simulink model "Task1_version5"  (R2021a)
settings: Solver=FixedStepAuto  StartTime=0.0  StopTime=0.05  FixedStep=1e-7  MaxStep=1e-7  RelTol=1e-3
values from neighbouring files (symbols this model uses):
  f0 = str2double(inputStr)    [PWM.m]
  fs = Switching_frequency(j)    [PWM.m]
  M = 1    [PWM.m]
  Mode = 1    [PWM.m]
libraries: simulink x4, spspowerguiLib x1
settings Model: OrderedModelArguments=off  Creator=es-mostafamoh111  LastModifiedBy=es-mostafamoh111
settings DataIOCC: ReturnWorkspaceOutputs=off

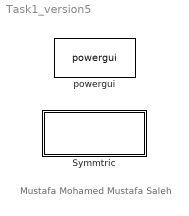
== system Task1_version5 ==
  note: Mustafa Mohamed Mustafa Saleh
  Symmtric : Subsystem
  powergui : spspowerguiLib/powergui  Priority=1  SimulationMode=Discrete  SampleTime=1e-7  frequency=60  Iterations=50  frequencyindice=0  Pbase=100e6  ErrMax=1e-4  UnitsV=kV  UnitsW=MW  buscounter=0  FunctionMessages=off  echomessages=off  EnableUseOfTLC=off  CurrentSourceSwitches=off  DisableSnubberDevices=off  DisableRonSwitches=off  DisableVfSwitches=off  DisplayEquations=off  AutomaticDiscreteSolvers=off  SolverType=Tustin/Backward Euler (TBE)  Interpol=off  ExternalGateDelay=off  methode=off  Ts=100  x0status=blocks  SPID=on  SwTol=0  HookPort=off  NonlinearTolerance=1e-4  nMaxIteration=100  ContinueOnMaxIteration=off  RestoreLinks=warning  ResistiveCurrentMeasurement=off  Frange=[0:2:500]  Ylog=off  Xlog=on  ShowGrid=off  save=off  variable=ZData  structure=0  ZoomFFT=off  StartTime=0.0  cycles=1  DisplayStyle=1  fundamental=60  FreqAxis=off  MaxFrequency=1000  frequencyindicesteady=1  RmsSteady=1  display=off

== system Task1_version5/Symmtric ==
  Symmetric DPWM1 : Subsystem
  Symmetric SPWM : Subsystem
  Symmetric SVM : Subsystem

== system Task1_version5/Symmtric/Symmetric DPWM1 ==
  DPWM max : Subsystem  Commented=on  TreatAsAtomicUnit=on
  DPWM min : Subsystem  Commented=on  TreatAsAtomicUnit=on
  DPWM1 : Subsystem
  Nature sine DPWM : Subsystem  Commented=on

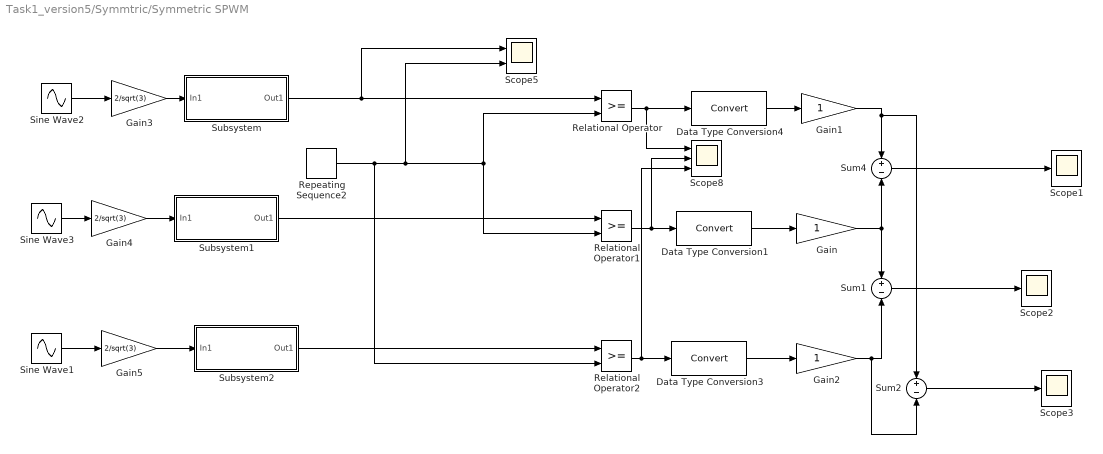
== system Task1_version5/Symmtric/Symmetric SPWM ==
  Data Type Conversion1 : DataTypeConversion
  Data Type Conversion3 : DataTypeConversion
  Data Type Conversion4 : DataTypeConversion
  Gain : Gain
  Gain1 : Gain  OutDataTypeStr=Inherit: Inherit via back propagation
  Gain2 : Gain
  Gain3 : Gain  Gain=2/sqrt(3)
  Gain4 : Gain  Gain=2/sqrt(3)
  Gain5 : Gain  Gain=2/sqrt(3)
  Relational Operator : RelationalOperator  OutDataTypeStr=boolean  RndMeth=Simplest
  Relational Operator1 : RelationalOperator  OutDataTypeStr=boolean  RndMeth=Simplest
  Relational Operator2 : RelationalOperator  OutDataTypeStr=boolean  RndMeth=Simplest
  Repeating Sequence2 : simulink/Sources/Repeating Sequence  rep_seq_t=[0 1/(4*fs) 2/(4*fs) 3/(4*fs) 1/fs ]  rep_seq_y=[1 0 -1 0 1]
  Scope1 : Scope
  Scope2 : Scope
  Scope3 : Scope
  Scope5 : Scope  NumInputPorts=2
  Scope8 : Scope  NumInputPorts=3
  Sine Wave1 : Sin  Amplitude=M  Frequency=f0*2*pi  Phase=2*pi/3  SampleTime=0
  Sine Wave2 : Sin  Amplitude=M  Frequency=f0*2*pi  SampleTime=0
  Sine Wave3 : Sin  Amplitude=M  Frequency=f0*2*pi  Phase=-2*pi/3  SampleTime=0
  Subsystem : Subsystem
  Subsystem1 : Subsystem
  Subsystem2 : Subsystem
  Sum1 : Sum  Inputs=+-
  Sum2 : Sum  Inputs=+-
  Sum4 : Sum  Inputs=+-
  wires:
  Gain/1 -> Sum4/2, Sum1/1
  Gain1/1 -> Sum2/1, Sum4/1
  Repeating Sequence2/1 -> Relational Operator2/2, Scope5/2, Relational Operator/2, Relational Operator1/2
  Subsystem/1(Out1) -> Scope5/1, Relational Operator/1
  Sine Wave2/1 -> Gain3/1
  Relational Operator1/1 -> Scope8/2, Data Type Conversion1/1
  Relational Operator/1 -> Scope8/1, Data Type Conversion4/1
  Sine Wave1/1 -> Gain5/1
  Data Type Conversion3/1 -> Gain2/1
  Relational Operator2/1 -> Scope8/3, Data Type Conversion3/1
  Data Type Conversion4/1 -> Gain1/1
  Data Type Conversion1/1 -> Gain/1
  Gain2/1 -> Sum2/2, Sum1/2
  Sine Wave3/1 -> Gain4/1
  Subsystem1/1(Out1) -> Relational Operator1/1
  Subsystem2/1(Out1) -> Relational Operator2/1
  Sum4/1 -> Scope1/1
  Sum1/1 -> Scope2/1
  Sum2/1 -> Scope3/1
  Gain3/1 -> Subsystem/1(In1)
  Gain4/1 -> Subsystem1/1(In1)
  Gain5/1 -> Subsystem2/1(In1)

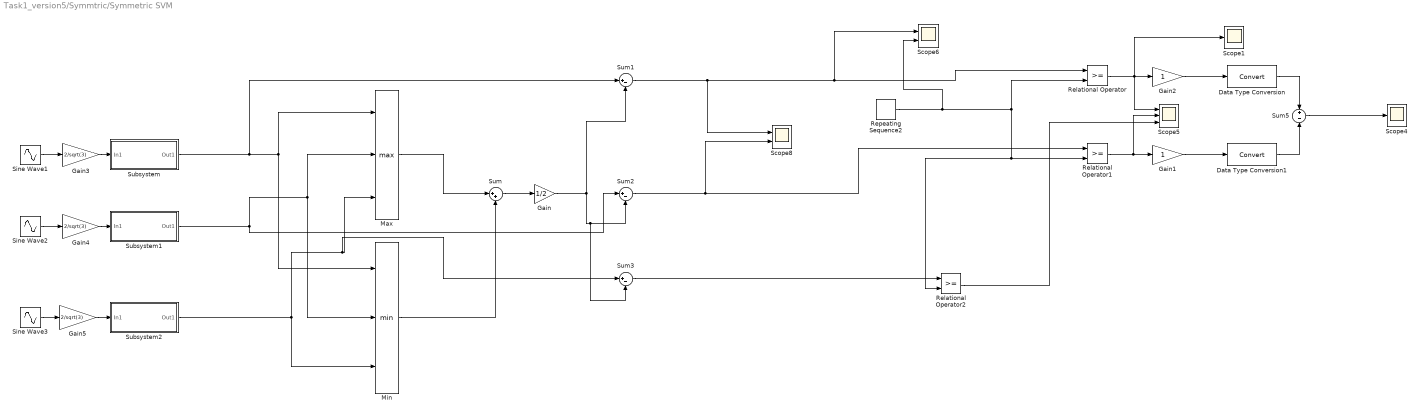
== system Task1_version5/Symmtric/Symmetric SVM ==
  Data Type Conversion : DataTypeConversion
  Data Type Conversion1 : DataTypeConversion
  Gain : Gain  Gain=1/2
  Gain1 : Gain
  Gain2 : Gain
  Gain3 : Gain  Gain=2/sqrt(3)
  Gain4 : Gain  Gain=2/sqrt(3)
  Gain5 : Gain  Gain=2/sqrt(3)
  Max : MinMax  Function=max  Inputs=3
  Min : MinMax  Inputs=3
  Relational Operator : RelationalOperator  OutDataTypeStr=boolean  RndMeth=Simplest
  Relational Operator1 : RelationalOperator  OutDataTypeStr=boolean  RndMeth=Simplest
  Relational Operator2 : RelationalOperator  OutDataTypeStr=boolean  RndMeth=Simplest
  Repeating Sequence2 : simulink/Sources/Repeating Sequence  rep_seq_t=[0 1/(4*fs) 2/(4*fs) 3/(4*fs) 1/fs ]  rep_seq_y=[1 0 -1 0 1]
  Scope1 : Scope
  Scope4 : Scope
  Scope5 : Scope  NumInputPorts=3
  Scope6 : Scope  NumInputPorts=2
  Scope8 : Scope  NumInputPorts=2
  Sine Wave1 : Sin  Amplitude=M  Frequency=f0*2*pi  SampleTime=0
  Sine Wave2 : Sin  Amplitude=M  Frequency=f0*2*pi  Phase=-2*pi/3  SampleTime=0
  Sine Wave3 : Sin  Amplitude=M  Frequency=f0*2*pi  Phase=2*pi/3  SampleTime=0
  Subsystem : Subsystem
  Subsystem1 : Subsystem
  Subsystem2 : Subsystem
  Sum : Sum  Inputs=|++
  Sum1 : Sum  Inputs=|+-
  Sum2 : Sum  Inputs=|+-
  Sum3 : Sum  Inputs=|+-
  Sum5 : Sum  Inputs=+-
  wires:
  Subsystem/1(Out1) -> Sum1/1, Min/1, Max/1
  Relational Operator/1 -> Scope1/1, Gain2/1, Scope5/1
  Repeating Sequence2/1 -> Scope6/2, Relational Operator/2, Relational Operator1/2, Relational Operator2/2
  Sum/1 -> Gain/1
  Subsystem1/1(Out1) -> Min/2, Max/2, Sum2/1
  Relational Operator1/1 -> Scope5/2, Gain1/1
  Gain/1 -> Sum2/2, Sum3/2, Sum1/2
  Max/1 -> Sum/1
  Gain1/1 -> Data Type Conversion1/1
  Min/1 -> Sum/2
  Data Type Conversion1/1 -> Sum5/2
  Data Type Conversion/1 -> Sum5/1
  Gain2/1 -> Data Type Conversion/1
  Subsystem2/1(Out1) -> Sum3/1, Max/3, Min/3
  Relational Operator2/1 -> Scope5/3
  Sum3/1 -> Relational Operator2/1
  Sum2/1 -> Relational Operator1/1, Scope8/2
  Sum1/1 -> Scope6/1, Relational Operator/1, Scope8/1
  Sine Wave1/1 -> Gain3/1
  Sine Wave2/1 -> Gain4/1
  Sine Wave3/1 -> Gain5/1
  Sum5/1 -> Scope4/1
  Gain3/1 -> Subsystem/1(In1)
  Gain4/1 -> Subsystem1/1(In1)
  Gain5/1 -> Subsystem2/1(In1)

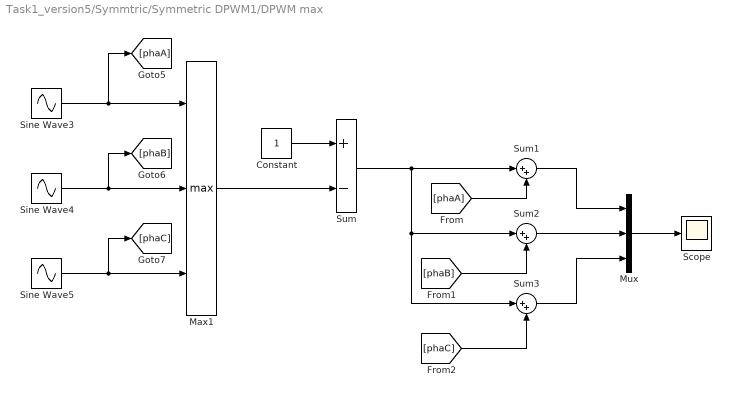
== system Task1_version5/Symmtric/Symmetric DPWM1/DPWM max ==
  Constant : Constant
  Max1 : MinMax  Function=max  Inputs=3
  Mux : Mux  Inputs=3
  Scope : Scope
  Sine Wave3 : Sin  Frequency=2*pi*f0  SampleTime=0
  Sine Wave4 : Sin  Frequency=2*pi*f0  Phase=-2*pi/3  SampleTime=0
  Sine Wave5 : Sin  Frequency=2*pi*f0  Phase=2*pi/3  SampleTime=0
  Sum : Sum  Inputs=+-
  Sum1 : Sum  Inputs=|++
  Sum2 : Sum  Inputs=|++
  Sum3 : Sum  Inputs=|++
  wires:
  Sine Wave4/1 -> [phaB], Max1/2
  Sine Wave3/1 -> [phaA], Max1/1
  Sine Wave5/1 -> [phaC], Max1/3
  [phaB] -> Sum2/2
  Sum/1 -> Sum2/1, Sum3/1, Sum1/1
  Sum3/1 -> Mux/3
  Sum1/1 -> Mux/1
  Sum2/1 -> Mux/2
  Mux/1 -> Scope/1
  [phaA] -> Sum1/2
  [phaC] -> Sum3/2
  Constant/1 -> Sum/1
  Max1/1 -> Sum/2

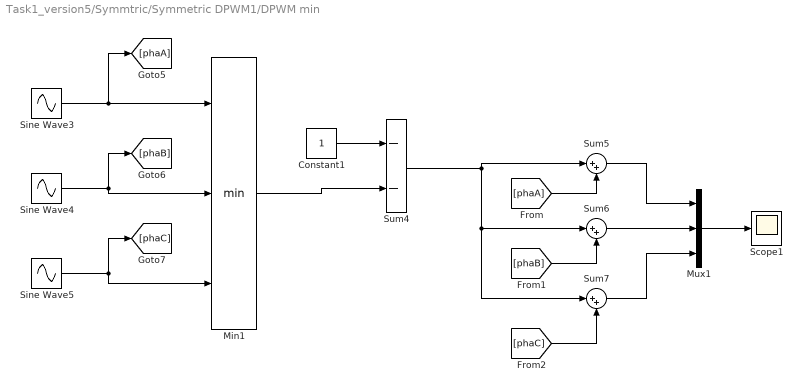
== system Task1_version5/Symmtric/Symmetric DPWM1/DPWM min ==
  Constant1 : Constant
  Min1 : MinMax  Inputs=3
  Mux1 : Mux  Inputs=3
  Scope1 : Scope
  Sine Wave3 : Sin  Frequency=2*pi*f0  SampleTime=0
  Sine Wave4 : Sin  Frequency=2*pi*f0  Phase=-2*pi/3  SampleTime=0
  Sine Wave5 : Sin  Frequency=2*pi*f0  Phase=2*pi/3  SampleTime=0
  Sum4 : Sum  Inputs=--
  Sum5 : Sum  Inputs=|++
  Sum6 : Sum  Inputs=|++
  Sum7 : Sum  Inputs=|++
  wires:
  Min1/1 -> Sum4/2
  Sine Wave4/1 -> [phaB], Min1/2
  Sine Wave3/1 -> [phaA], Min1/1
  Sine Wave5/1 -> [phaC], Min1/3
  [phaA] -> Sum5/2
  [phaB] -> Sum6/2
  Mux1/1 -> Scope1/1
  Sum7/1 -> Mux1/3
  [phaC] -> Sum7/2
  Sum5/1 -> Mux1/1
  Sum6/1 -> Mux1/2
  Constant1/1 -> Sum4/1
  Sum4/1 -> Sum5/1, Sum6/1, Sum7/1

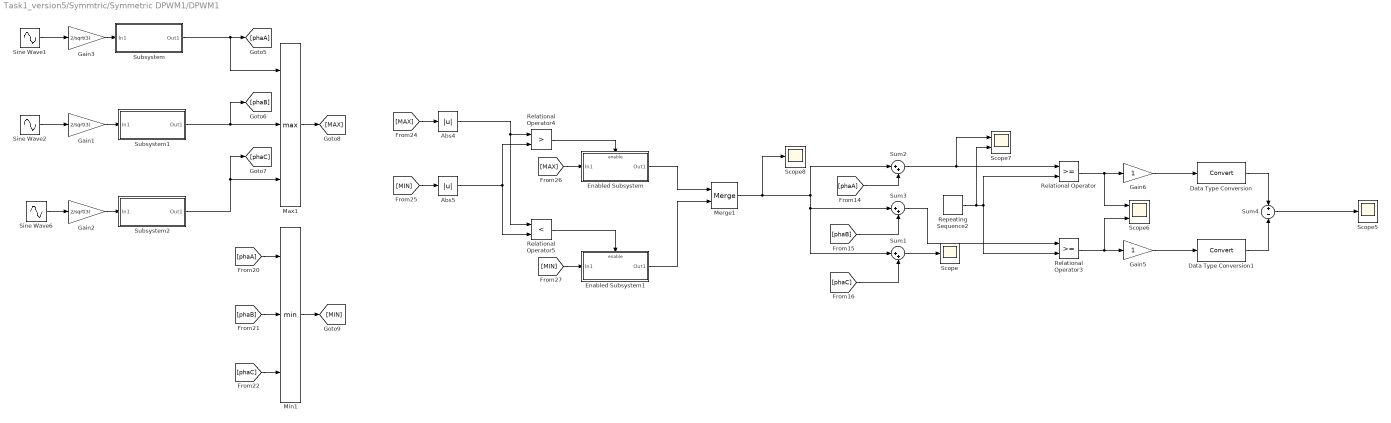
== system Task1_version5/Symmtric/Symmetric DPWM1/DPWM1 ==
  Abs4 : Abs
  Abs5 : Abs
  Data Type Conversion : DataTypeConversion
  Data Type Conversion1 : DataTypeConversion
  Enabled Subsystem : Subsystem  TreatAsAtomicUnit=on
  Enabled Subsystem1 : Subsystem  TreatAsAtomicUnit=on
  Gain1 : Gain  Gain=2/sqrt(3)
  Gain2 : Gain  Gain=2/sqrt(3)
  Gain3 : Gain  Gain=2/sqrt(3)
  Gain5 : Gain
  Gain6 : Gain
  Max1 : MinMax  Function=max  Inputs=3
  Merge1 : Merge
  Min1 : MinMax  Inputs=3
  Relational Operator : RelationalOperator  OutDataTypeStr=boolean  RndMeth=Simplest
  Relational Operator3 : RelationalOperator  OutDataTypeStr=boolean  RndMeth=Simplest
  Relational Operator4 : RelationalOperator  Operator=>  OutDataTypeStr=boolean  RndMeth=Simplest
  Relational Operator5 : RelationalOperator  Operator=<  OutDataTypeStr=boolean  RndMeth=Simplest
  Repeating Sequence2 : simulink/Sources/Repeating Sequence  rep_seq_t=[0 1/(4*fs) 2/(4*fs) 3/(4*fs) 1/fs ]  rep_seq_y=[1 0 -1 0 1]
  Scope : Scope
  Scope5 : Scope
  Scope6 : Scope  NumInputPorts=2
  Scope7 : Scope  NumInputPorts=2
  Scope8 : Scope
  Sine Wave1 : Sin  Amplitude=M  Frequency=f0*2*pi  SampleTime=0
  Sine Wave2 : Sin  Amplitude=M  Frequency=f0*2*pi  Phase=-2*pi/3  SampleTime=0
  Sine Wave6 : Sin  Amplitude=M  Frequency=f0*2*pi  Phase=2*pi/3  SampleTime=0
  Subsystem : Subsystem
  Subsystem1 : Subsystem
  Subsystem2 : Subsystem
  Sum1 : Sum  Inputs=|++
  Sum2 : Sum  Inputs=|++
  Sum3 : Sum  Inputs=|++
  Sum4 : Sum  Inputs=+-
  wires:
  Sine Wave1/1 -> Gain3/1
  Sine Wave6/1 -> Gain2/1
  Sine Wave2/1 -> Gain1/1
  Max1/1 -> [MAX]
  [MAX] -> Abs4/1
  [phaB] -> Min1/2
  Subsystem/1(Out1) -> Max1/1, [phaA]
  Min1/1 -> [MIN]
  [phaA] -> Min1/1
  [MIN] -> Enabled Subsystem1/1(In1)
  Abs5/1 -> Relational Operator5/2, Relational Operator4/2
  Subsystem2/1(Out1) -> [phaC], Max1/3
  [phaB] -> Sum3/2
  [phaC] -> Min1/3
  Subsystem1/1(Out1) -> [phaB], Max1/2
  Relational Operator4/1 -> Enabled Subsystem/Enable
  Enabled Subsystem1/1(Out1) -> Merge1/2
  Merge1/1 -> Sum2/1, Sum3/1, Sum1/1, Scope8/1
  Abs4/1 -> Relational Operator4/1, Relational Operator5/1
  [phaC] -> Sum1/2
  [MAX] -> Enabled Subsystem/1(In1)
  Enabled Subsystem/1(Out1) -> Merge1/1
  Relational Operator5/1 -> Enabled Subsystem1/Enable
  [MIN] -> Abs5/1
  [phaA] -> Sum2/2
  Repeating Sequence2/1 -> Scope7/2, Relational Operator/2, Relational Operator3/2
  Gain5/1 -> Data Type Conversion1/1
  Data Type Conversion1/1 -> Sum4/2
  Relational Operator3/1 -> Scope6/2, Gain5/1
  Gain6/1 -> Data Type Conversion/1
  Data Type Conversion/1 -> Sum4/1
  Relational Operator/1 -> Gain6/1, Scope6/1
  Sum2/1 -> Scope7/1, Relational Operator/1
  Sum3/1 -> Relational Operator3/1
  Sum1/1 -> Scope/1
  Sum4/1 -> Scope5/1
  Gain3/1 -> Subsystem/1(In1)
  Gain1/1 -> Subsystem1/1(In1)
  Gain2/1 -> Subsystem2/1(In1)

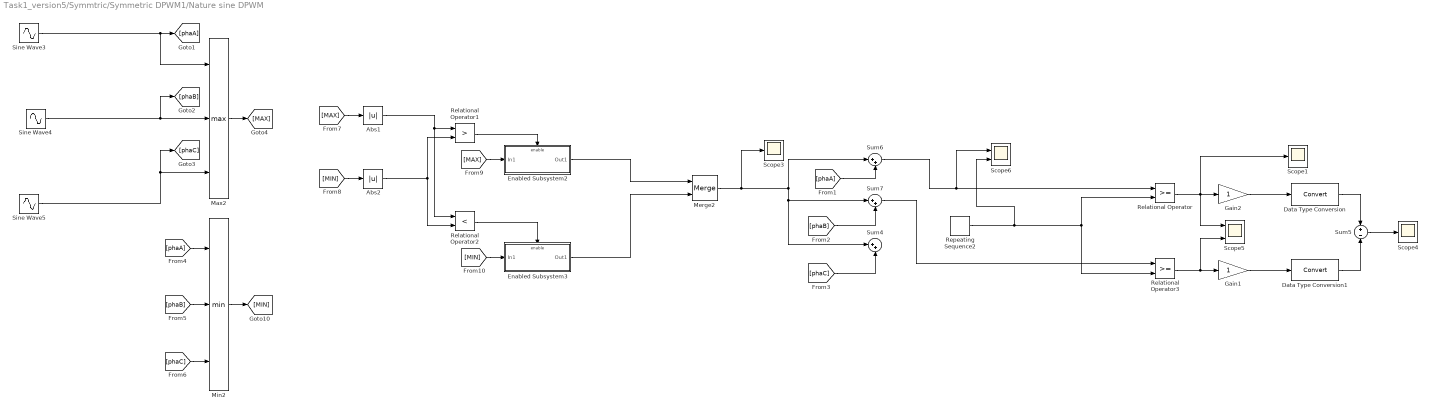
== system Task1_version5/Symmtric/Symmetric DPWM1/Nature sine DPWM ==
  Abs1 : Abs
  Abs2 : Abs
  Data Type Conversion : DataTypeConversion
  Data Type Conversion1 : DataTypeConversion
  Enabled Subsystem2 : Subsystem  TreatAsAtomicUnit=on
  Enabled Subsystem3 : Subsystem  TreatAsAtomicUnit=on
  Gain1 : Gain
  Gain2 : Gain
  Max2 : MinMax  Function=max  Inputs=3
  Merge2 : Merge
  Min2 : MinMax  Inputs=3
  Relational Operator : RelationalOperator  OutDataTypeStr=boolean  RndMeth=Simplest
  Relational Operator1 : RelationalOperator  Operator=>  OutDataTypeStr=boolean  RndMeth=Simplest
  Relational Operator2 : RelationalOperator  Operator=<  OutDataTypeStr=boolean  RndMeth=Simplest
  Relational Operator3 : RelationalOperator  OutDataTypeStr=boolean  RndMeth=Simplest
  Repeating Sequence2 : simulink/Sources/Repeating Sequence  rep_seq_t=[0 1/(4*fs) 2/(4*fs) 3/(4*fs) 1/fs ]  rep_seq_y=[1 0 -1 0 1]
  Scope1 : Scope
  Scope3 : Scope
  Scope4 : Scope
  Scope5 : Scope  NumInputPorts=2
  Scope6 : Scope  NumInputPorts=2
  Sine Wave3 : Sin  Amplitude=M  Frequency=f0*2*pi  SampleTime=0
  Sine Wave4 : Sin  Amplitude=M  Frequency=f0*2*pi  Phase=-2*pi/3  SampleTime=0
  Sine Wave5 : Sin  Amplitude=M  Frequency=f0*2*pi  Phase=2*pi/3  SampleTime=0
  Sum4 : Sum  Inputs=|++
  Sum5 : Sum  Inputs=+-
  Sum6 : Sum  Inputs=|++
  Sum7 : Sum  Inputs=|++
  wires:
  Abs2/1 -> Relational Operator2/2, Relational Operator1/2
  Min2/1 -> [MIN]
  Sine Wave5/1 -> [phaC], Max2/3
  [phaA] -> Min2/1
  Sine Wave4/1 -> [phaB], Max2/2
  [MIN] -> Enabled Subsystem3/1(In1)
  Sine Wave3/1 -> [phaA], Max2/1
  Merge2/1 -> Sum6/1, Sum7/1, Sum4/1, Scope3/1
  [phaC] -> Min2/3
  Enabled Subsystem3/1(Out1) -> Merge2/2
  Relational Operator2/1 -> Enabled Subsystem3/Enable
  Relational Operator1/1 -> Enabled Subsystem2/Enable
  Enabled Subsystem2/1(Out1) -> Merge2/1
  [phaB] -> Sum7/2
  [phaC] -> Sum4/2
  [MAX] -> Abs1/1
  [MAX] -> Enabled Subsystem2/1(In1)
  Abs1/1 -> Relational Operator1/1, Relational Operator2/1
  [phaA] -> Sum6/2
  [MIN] -> Abs2/1
  [phaB] -> Min2/2
  Max2/1 -> [MAX]
  Data Type Conversion/1 -> Sum5/1
  Gain2/1 -> Data Type Conversion/1
  Relational Operator3/1 -> Scope5/2, Gain1/1
  Sum5/1 -> Scope4/1
  Repeating Sequence2/1 -> Scope6/2, Relational Operator/2, Relational Operator3/2
  Relational Operator/1 -> Scope1/1, Gain2/1, Scope5/1
  Data Type Conversion1/1 -> Sum5/2
  Gain1/1 -> Data Type Conversion1/1
  Sum6/1 -> Scope6/1, Relational Operator/1
  Sum7/1 -> Relational Operator3/1

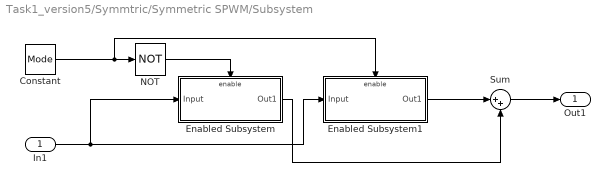
== system Task1_version5/Symmtric/Symmetric SPWM/Subsystem ==
  In1 : Inport
  Constant : Constant  Value=Mode
  Enabled Subsystem : Subsystem  TreatAsAtomicUnit=on
  Enabled Subsystem1 : Subsystem  TreatAsAtomicUnit=on
  NOT : Logic  Operator=NOT  IconShape=distinctive  AllPortsSameDT=off  OutDataTypeStr=boolean
  Sum : Sum  Inputs=|++
  Out1 : Outport
  wires:
  In1/1 -> Enabled Subsystem1/1(Input), Enabled Subsystem/1(Input)
  Constant/1 -> NOT/1, Enabled Subsystem1/Enable
  NOT/1 -> Enabled Subsystem/Enable
  Enabled Subsystem1/1(Out1) -> Sum/1
  Enabled Subsystem/1(Out1) -> Sum/2
  Sum/1 -> Out1/1

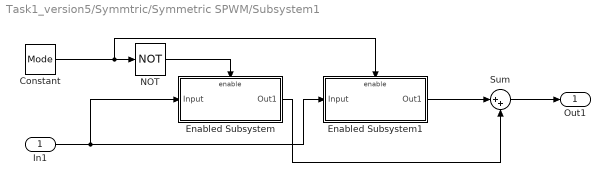
== system Task1_version5/Symmtric/Symmetric SPWM/Subsystem1 ==
  In1 : Inport
  Constant : Constant  Value=Mode
  Enabled Subsystem : Subsystem  TreatAsAtomicUnit=on
  Enabled Subsystem1 : Subsystem  TreatAsAtomicUnit=on
  NOT : Logic  Operator=NOT  IconShape=distinctive  AllPortsSameDT=off  OutDataTypeStr=boolean
  Sum : Sum  Inputs=|++
  Out1 : Outport
  wires:
  Sum/1 -> Out1/1
  Enabled Subsystem/1(Out1) -> Sum/2
  Enabled Subsystem1/1(Out1) -> Sum/1
  NOT/1 -> Enabled Subsystem/Enable
  Constant/1 -> Enabled Subsystem1/Enable, NOT/1
  In1/1 -> Enabled Subsystem/1(Input), Enabled Subsystem1/1(Input)

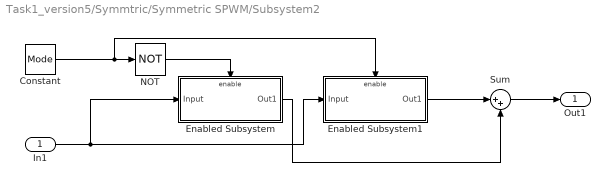
== system Task1_version5/Symmtric/Symmetric SPWM/Subsystem2 ==
  In1 : Inport
  Constant : Constant  Value=Mode
  Enabled Subsystem : Subsystem  TreatAsAtomicUnit=on
  Enabled Subsystem1 : Subsystem  TreatAsAtomicUnit=on
  NOT : Logic  Operator=NOT  IconShape=distinctive  AllPortsSameDT=off  OutDataTypeStr=boolean
  Sum : Sum  Inputs=|++
  Out1 : Outport
  wires:
  In1/1 -> Enabled Subsystem1/1(Input), Enabled Subsystem/1(Input)
  Constant/1 -> NOT/1, Enabled Subsystem1/Enable
  NOT/1 -> Enabled Subsystem/Enable
  Enabled Subsystem1/1(Out1) -> Sum/1
  Enabled Subsystem/1(Out1) -> Sum/2
  Sum/1 -> Out1/1

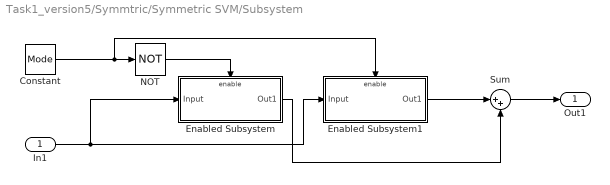
== system Task1_version5/Symmtric/Symmetric SVM/Subsystem ==
  In1 : Inport
  Constant : Constant  Value=Mode
  Enabled Subsystem : Subsystem  TreatAsAtomicUnit=on
  Enabled Subsystem1 : Subsystem  TreatAsAtomicUnit=on
  NOT : Logic  Operator=NOT  IconShape=distinctive  AllPortsSameDT=off  OutDataTypeStr=boolean
  Sum : Sum  Inputs=|++
  Out1 : Outport
  wires:
  In1/1 -> Enabled Subsystem1/1(Input), Enabled Subsystem/1(Input)
  Constant/1 -> NOT/1, Enabled Subsystem1/Enable
  NOT/1 -> Enabled Subsystem/Enable
  Enabled Subsystem1/1(Out1) -> Sum/1
  Enabled Subsystem/1(Out1) -> Sum/2
  Sum/1 -> Out1/1

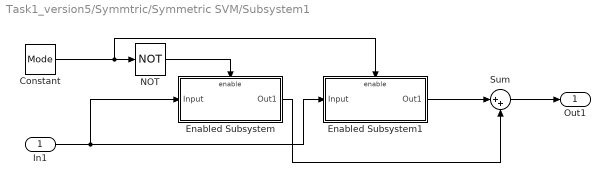
== system Task1_version5/Symmtric/Symmetric SVM/Subsystem1 ==
  In1 : Inport
  Constant : Constant  Value=Mode
  Enabled Subsystem : Subsystem  TreatAsAtomicUnit=on
  Enabled Subsystem1 : Subsystem  TreatAsAtomicUnit=on
  NOT : Logic  Operator=NOT  IconShape=distinctive  AllPortsSameDT=off  OutDataTypeStr=boolean
  Sum : Sum  Inputs=|++
  Out1 : Outport
  wires:
  Sum/1 -> Out1/1
  Enabled Subsystem/1(Out1) -> Sum/2
  Enabled Subsystem1/1(Out1) -> Sum/1
  NOT/1 -> Enabled Subsystem/Enable
  Constant/1 -> Enabled Subsystem1/Enable, NOT/1
  In1/1 -> Enabled Subsystem/1(Input), Enabled Subsystem1/1(Input)

== system Task1_version5/Symmtric/Symmetric SVM/Subsystem2 ==
  In1 : Inport
  Constant : Constant  Value=Mode
  Enabled Subsystem : Subsystem  TreatAsAtomicUnit=on
  Enabled Subsystem1 : Subsystem  TreatAsAtomicUnit=on
  NOT : Logic  Operator=NOT  IconShape=distinctive  AllPortsSameDT=off  OutDataTypeStr=boolean
  Sum : Sum  Inputs=|++
  Out1 : Outport
  wires:
  In1/1 -> Enabled Subsystem1/1(Input), Enabled Subsystem/1(Input)
  Constant/1 -> NOT/1, Enabled Subsystem1/Enable
  NOT/1 -> Enabled Subsystem/Enable
  Enabled Subsystem1/1(Out1) -> Sum/1
  Enabled Subsystem/1(Out1) -> Sum/2
  Sum/1 -> Out1/1

== system Task1_version5/Symmtric/Symmetric DPWM1/DPWM1/Enabled Subsystem ==
  In1 : Inport
  Enable : EnablePort
  Constant : Constant
  Scope : Scope
  Sum : Sum  Inputs=+-
  Out1 : Outport
  wires:
  Sum/1 -> Out1/1, Scope/1
  In1/1 -> Sum/2
  Constant/1 -> Sum/1

== system Task1_version5/Symmtric/Symmetric DPWM1/DPWM1/Enabled Subsystem1 ==
  In1 : Inport
  Enable : EnablePort
  Constant : Constant
  Scope : Scope
  Sum : Sum  Inputs=--
  Out1 : Outport
  wires:
  In1/1 -> Sum/2
  Constant/1 -> Sum/1
  Sum/1 -> Out1/1, Scope/1

== system Task1_version5/Symmtric/Symmetric DPWM1/DPWM1/Subsystem ==
  In1 : Inport
  Constant : Constant  Value=Mode
  Enabled Subsystem : Subsystem  TreatAsAtomicUnit=on
  Enabled Subsystem1 : Subsystem  TreatAsAtomicUnit=on
  NOT : Logic  Operator=NOT  IconShape=distinctive  AllPortsSameDT=off  OutDataTypeStr=boolean
  Sum : Sum  Inputs=|++
  Out1 : Outport
  wires:
  In1/1 -> Enabled Subsystem1/1(Input), Enabled Subsystem/1(Input)
  Constant/1 -> NOT/1, Enabled Subsystem1/Enable
  NOT/1 -> Enabled Subsystem/Enable
  Enabled Subsystem1/1(Out1) -> Sum/1
  Enabled Subsystem/1(Out1) -> Sum/2
  Sum/1 -> Out1/1

== system Task1_version5/Symmtric/Symmetric DPWM1/DPWM1/Subsystem1 ==
  In1 : Inport
  Constant : Constant  Value=Mode
  Enabled Subsystem : Subsystem  TreatAsAtomicUnit=on
  Enabled Subsystem1 : Subsystem  TreatAsAtomicUnit=on
  NOT : Logic  Operator=NOT  IconShape=distinctive  AllPortsSameDT=off  OutDataTypeStr=boolean
  Sum : Sum  Inputs=|++
  Out1 : Outport
  wires:
  Sum/1 -> Out1/1
  Enabled Subsystem/1(Out1) -> Sum/2
  Enabled Subsystem1/1(Out1) -> Sum/1
  NOT/1 -> Enabled Subsystem/Enable
  Constant/1 -> Enabled Subsystem1/Enable, NOT/1
  In1/1 -> Enabled Subsystem/1(Input), Enabled Subsystem1/1(Input)

== system Task1_version5/Symmtric/Symmetric DPWM1/DPWM1/Subsystem2 ==
  In1 : Inport
  Constant : Constant  Value=Mode
  Enabled Subsystem : Subsystem  TreatAsAtomicUnit=on
  Enabled Subsystem1 : Subsystem  TreatAsAtomicUnit=on
  NOT : Logic  Operator=NOT  IconShape=distinctive  AllPortsSameDT=off  OutDataTypeStr=boolean
  Sum : Sum  Inputs=|++
  Out1 : Outport
  wires:
  In1/1 -> Enabled Subsystem1/1(Input), Enabled Subsystem/1(Input)
  Constant/1 -> NOT/1, Enabled Subsystem1/Enable
  NOT/1 -> Enabled Subsystem/Enable
  Enabled Subsystem1/1(Out1) -> Sum/1
  Enabled Subsystem/1(Out1) -> Sum/2
  Sum/1 -> Out1/1

== system Task1_version5/Symmtric/Symmetric DPWM1/Nature sine DPWM/Enabled Subsystem2 ==
  In1 : Inport
  Enable : EnablePort
  Constant : Constant
  Scope : Scope
  Sum : Sum  Inputs=+-
  Out1 : Outport
  wires:
  Sum/1 -> Out1/1, Scope/1
  In1/1 -> Sum/2
  Constant/1 -> Sum/1

== system Task1_version5/Symmtric/Symmetric DPWM1/Nature sine DPWM/Enabled Subsystem3 ==
  In1 : Inport
  Enable : EnablePort
  Constant : Constant
  Scope : Scope
  Sum : Sum  Inputs=--
  Out1 : Outport
  wires:
  In1/1 -> Sum/2
  Constant/1 -> Sum/1
  Sum/1 -> Out1/1, Scope/1

== system Task1_version5/Symmtric/Symmetric SPWM/Subsystem/Enabled Subsystem ==
  Input : Inport
  Enable : EnablePort
  Zero-Order Hold : ZeroOrderHold  SampleTime=1/(fs)
  Out1 : Outport
  wires:
  Input/1 -> Zero-Order Hold/1
  Zero-Order Hold/1 -> Out1/1

== system Task1_version5/Symmtric/Symmetric SPWM/Subsystem/Enabled Subsystem1 ==
  Input : Inport
  Enable : EnablePort
  Zero-Order Hold1 : ZeroOrderHold  SampleTime=1/(2*fs)
  Out1 : Outport
  wires:
  Zero-Order Hold1/1 -> Out1/1
  Input/1 -> Zero-Order Hold1/1

== system Task1_version5/Symmtric/Symmetric SPWM/Subsystem1/Enabled Subsystem ==
  Input : Inport
  Enable : EnablePort
  Zero-Order Hold : ZeroOrderHold  SampleTime=1/(fs)
  Out1 : Outport
  wires:
  Zero-Order Hold/1 -> Out1/1
  Input/1 -> Zero-Order Hold/1

== system Task1_version5/Symmtric/Symmetric SPWM/Subsystem1/Enabled Subsystem1 ==
  Input : Inport
  Enable : EnablePort
  Zero-Order Hold1 : ZeroOrderHold  SampleTime=1/(2*fs)
  Out1 : Outport
  wires:
  Input/1 -> Zero-Order Hold1/1
  Zero-Order Hold1/1 -> Out1/1

== system Task1_version5/Symmtric/Symmetric SPWM/Subsystem2/Enabled Subsystem ==
  Input : Inport
  Enable : EnablePort
  Zero-Order Hold : ZeroOrderHold  SampleTime=1/(fs)
  Out1 : Outport
  wires:
  Input/1 -> Zero-Order Hold/1
  Zero-Order Hold/1 -> Out1/1

== system Task1_version5/Symmtric/Symmetric SPWM/Subsystem2/Enabled Subsystem1 ==
  Input : Inport
  Enable : EnablePort
  Zero-Order Hold1 : ZeroOrderHold  SampleTime=1/(2*fs)
  Out1 : Outport
  wires:
  Zero-Order Hold1/1 -> Out1/1
  Input/1 -> Zero-Order Hold1/1

== system Task1_version5/Symmtric/Symmetric SVM/Subsystem/Enabled Subsystem ==
  Input : Inport
  Enable : EnablePort
  Zero-Order Hold : ZeroOrderHold  SampleTime=1/(fs)
  Out1 : Outport
  wires:
  Input/1 -> Zero-Order Hold/1
  Zero-Order Hold/1 -> Out1/1

== system Task1_version5/Symmtric/Symmetric SVM/Subsystem/Enabled Subsystem1 ==
  Input : Inport
  Enable : EnablePort
  Zero-Order Hold1 : ZeroOrderHold  SampleTime=1/(2*fs)
  Out1 : Outport
  wires:
  Zero-Order Hold1/1 -> Out1/1
  Input/1 -> Zero-Order Hold1/1

== system Task1_version5/Symmtric/Symmetric SVM/Subsystem1/Enabled Subsystem ==
  Input : Inport
  Enable : EnablePort
  Zero-Order Hold : ZeroOrderHold  SampleTime=1/(fs)
  Out1 : Outport
  wires:
  Zero-Order Hold/1 -> Out1/1
  Input/1 -> Zero-Order Hold/1

== system Task1_version5/Symmtric/Symmetric SVM/Subsystem1/Enabled Subsystem1 ==
  Input : Inport
  Enable : EnablePort
  Zero-Order Hold1 : ZeroOrderHold  SampleTime=1/(2*fs)
  Out1 : Outport
  wires:
  Input/1 -> Zero-Order Hold1/1
  Zero-Order Hold1/1 -> Out1/1

== system Task1_version5/Symmtric/Symmetric SVM/Subsystem2/Enabled Subsystem ==
  Input : Inport
  Enable : EnablePort
  Zero-Order Hold : ZeroOrderHold  SampleTime=1/(fs)
  Out1 : Outport
  wires:
  Input/1 -> Zero-Order Hold/1
  Zero-Order Hold/1 -> Out1/1

== system Task1_version5/Symmtric/Symmetric SVM/Subsystem2/Enabled Subsystem1 ==
  Input : Inport
  Enable : EnablePort
  Zero-Order Hold1 : ZeroOrderHold  SampleTime=1/(2*fs)
  Out1 : Outport
  wires:
  Zero-Order Hold1/1 -> Out1/1
  Input/1 -> Zero-Order Hold1/1

== system Task1_version5/Symmtric/Symmetric DPWM1/DPWM1/Subsystem/Enabled Subsystem ==
  Input : Inport
  Enable : EnablePort
  Zero-Order Hold : ZeroOrderHold  SampleTime=1/(fs)
  Out1 : Outport
  wires:
  Input/1 -> Zero-Order Hold/1
  Zero-Order Hold/1 -> Out1/1

== system Task1_version5/Symmtric/Symmetric DPWM1/DPWM1/Subsystem/Enabled Subsystem1 ==
  Input : Inport
  Enable : EnablePort
  Zero-Order Hold1 : ZeroOrderHold  SampleTime=1/(2*fs)
  Out1 : Outport
  wires:
  Zero-Order Hold1/1 -> Out1/1
  Input/1 -> Zero-Order Hold1/1

== system Task1_version5/Symmtric/Symmetric DPWM1/DPWM1/Subsystem1/Enabled Subsystem ==
  Input : Inport
  Enable : EnablePort
  Zero-Order Hold : ZeroOrderHold  SampleTime=1/(fs)
  Out1 : Outport
  wires:
  Zero-Order Hold/1 -> Out1/1
  Input/1 -> Zero-Order Hold/1

== system Task1_version5/Symmtric/Symmetric DPWM1/DPWM1/Subsystem1/Enabled Subsystem1 ==
  Input : Inport
  Enable : EnablePort
  Zero-Order Hold1 : ZeroOrderHold  SampleTime=1/(2*fs)
  Out1 : Outport
  wires:
  Input/1 -> Zero-Order Hold1/1
  Zero-Order Hold1/1 -> Out1/1

== system Task1_version5/Symmtric/Symmetric DPWM1/DPWM1/Subsystem2/Enabled Subsystem ==
  Input : Inport
  Enable : EnablePort
  Zero-Order Hold : ZeroOrderHold  SampleTime=1/(fs)
  Out1 : Outport
  wires:
  Input/1 -> Zero-Order Hold/1
  Zero-Order Hold/1 -> Out1/1

== system Task1_version5/Symmtric/Symmetric DPWM1/DPWM1/Subsystem2/Enabled Subsystem1 ==
  Input : Inport
  Enable : EnablePort
  Zero-Order Hold1 : ZeroOrderHold  SampleTime=1/(2*fs)
  Out1 : Outport
  wires:
  Zero-Order Hold1/1 -> Out1/1
  Input/1 -> Zero-Order Hold1/1
